simulink model "LINEFOLLOW_90_DATA_READING"  (R2023a)
settings: Solver=FixedStepDiscrete  StartTime=0.0  StopTime=250  FixedStep=0.01  RelTol=1e-3
model workspace (MAT data in the model file):
  data = 0
undefined symbols (not defined in the file or in its folder): axleLength, InputPWM, ticksPerRot, wheelR, WheelSpeed
libraries: mobileRoboticsTrainingLib x7, simulink_extras x1
settings Model: SimulationMode=accelerator  PacingRate=18  Creator=nuvitdemirtas  LastModifiedBy=nuvitdemirtas

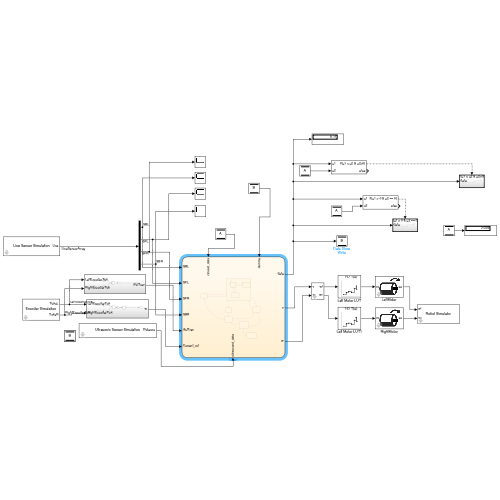
[thumbnail: Simulink's stored preview of the top-level diagram]
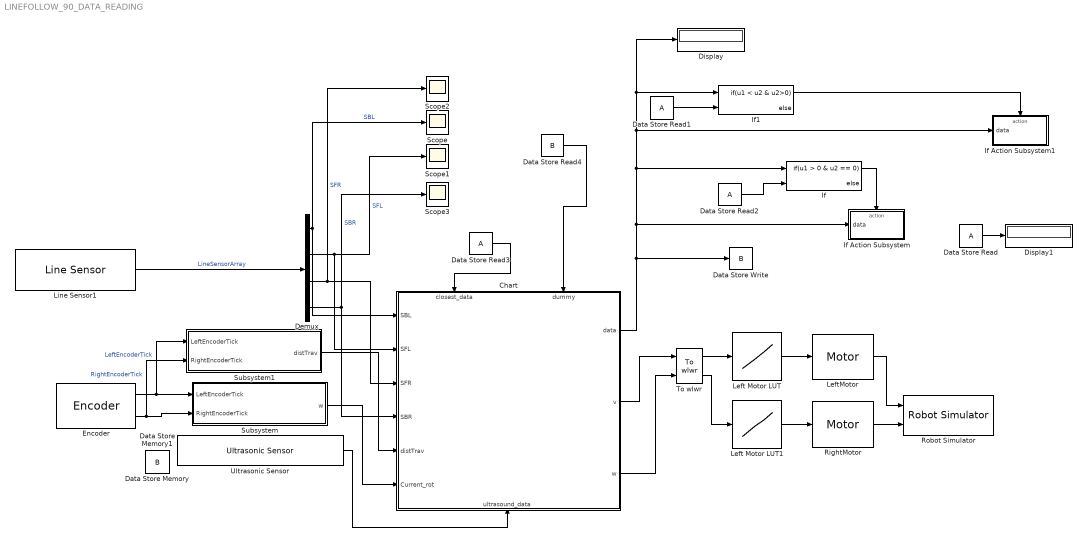
== system LINEFOLLOW_90_DATA_READING ==
  Chart : Stateflow chart  TreatAsAtomicUnit=on
      settings: PortSchema="{\"entries\":[{\"content\":{\"sides\":[{\"content\":{\"connectorIds\":[\"In5\",\"In3\",\"In2\",\"In4\",\"In7\",\"In6\"]},\"type\":\"ConnectorPlacement.EquallySpacedRectSide\",\"uuid\":\"3b08c9f5-f3e7-4190-8c9e-e5c4b273b76c\"},{\"content\":{\"connectorIds\":[\"Out3\",\"Out2\",\"Out1\"],\"side\":\"RIGHT\"},\"type\":\"ConnectorPlacement.EquallySpacedRectSide\",\"uuid\":\"91158a50-9984-4409-9676-111dc7610217\"},{\"content\":{\"connectorIds\":[\"In8\",\"In9\"],\"side\":\"TOP\"},\"type\":\"ConnectorPlacement.EquallySpacedRectSide\",\"uuid\":\"e43f7616-6a00-4e82-aaba-e999a0c0a235\"},{\"content\":{\"connectorIds\":[\"In1\"],\"side\":\"BOTTOM\"},\"type\":\"ConnectorPlacement.EquallySpacedRectSide\",\"uuid\":\"5780565f-9fed-471c-a43c-eef749218091\"}]},\"type\":\"ConnectorPlacement.EquallySpacedConnector\",\"uuid\":\"4b7d5f21-cf1e-4123-a6bd-16491044a199\"}],\"packageUris\":[\"http://schema.mathworks.com/mf0/Connector/R2020b\"],\"version\":\"1.0\"}"
  Data Store Read{,1..3} (4 alike) : DataStoreRead  IndexOptions=Index vector (dialog)  Indices=1  OutputSizes=1
  Data Store Read4 : DataStoreRead  DataStoreName=B  IndexOptions=Index vector (dialog)  Indices=1  OutputSizes=1
  Data Store Write : DataStoreWrite  DataStoreName=B  IndexOptions=Index vector (dialog)  Indices=1  OutputSizes=1
  Data Store Memory : DataStoreMemory  WriteAfterWriteMsg=warning  ShowAdditionalParam=off
  Data Store Memory1 : DataStoreMemory  DataStoreName=B  WriteAfterWriteMsg=warning  ShowAdditionalParam=off
  Demux : Demux
  Display : Display
  Display1 : Display
  Encoder : mobileRoboticsTrainingLib/Encoder  axleLength=axleLength  wheelR=wheelR  ticksPerRot=ticksPerRot
      settings: SourceProductName=Mobile Robotics Training Library
  If : If  NumInputs=2  IfExpression=u1 > 0 & u2 == 0
  If Action Subsystem : Subsystem  TreatAsAtomicUnit=on
  If Action Subsystem1 : Subsystem  TreatAsAtomicUnit=on
  If1 : If  NumInputs=2  IfExpression=u1 < u2 & u2>0
  Left Motor LUT : Lookup_n-D  NumberOfTableDimensions=1  BreakpointsForDimension1=WheelSpeed  Table=InputPWM  InterpMethod=Nearest  ExtrapMethod=Clip  InternalRulePriority=Speed  RndMeth=Simplest
  Left Motor LUT1 : Lookup_n-D  NumberOfTableDimensions=1  BreakpointsForDimension1=WheelSpeed  Table=InputPWM  InterpMethod=Nearest  ExtrapMethod=Clip  InternalRulePriority=Speed  RndMeth=Simplest
  LeftMotor : mobileRoboticsTrainingLib/Motor  motorPlant=wheelMotorModel  sensorType=Speed
      settings: SourceProductName=Mobile Robotics Training Library
  Line Sensor1 : mobileRoboticsTrainingLib/Line Sensor  mapVariable=mapForSim  envVal=1  lineVal=0  sensOff=[0.0643 0.0354; 0.0675 0.005; 0.0675 -0.005; 0.0643 -0.0354]
      link override Switch: Threshold=0
      settings: SourceProductName=Mobile Robotics Training Library
  RightMotor : mobileRoboticsTrainingLib/Motor  motorPlant=wheelMotorModel  sensorType=Speed
      settings: SourceProductName=Mobile Robotics Training Library
  Robot Simulator : mobileRoboticsTrainingLib/Robot Simulator  Priority=99  mapVar=mapForSim  startX=1.0088  startY=3.1003  startTheta=90  axleLength=axleLength  wheelR=wheelR
  Scope{,1..3} (4 alike) : Scope
  Subsystem : Subsystem
  Subsystem1 : Subsystem
  To wlwr : mobileRoboticsTrainingLib/To wlwr  axleLength=0.1  wheelR=0.05
  Ultrasonic Sensor : mobileRoboticsTrainingLib/Ultrasonic Sensor  mapVar=mapForSim  maxSenRange=4  minSenRange=0.02  senRes=0.003  sensOff=[0.1 0]
      settings: SourceProductName=Mobile Robotics Training Library
  wires:
  RightMotor/1 -> Robot Simulator/2
  LeftMotor/1 -> Robot Simulator/1
  To wlwr/2 -> Left Motor LUT1/1
  To wlwr/1 -> Left Motor LUT/1
  Chart/1(w) -> To wlwr/2
  Ultrasonic Sensor/1 -> Chart/1(ultrasound_data)
  Demux/4 -> Scope3/1, Chart/4(SBR)  "SBR"
  Encoder/2 -> Subsystem1/2(RightEncoderTick), Subsystem/2(RightEncoderTick)  "RightEncoderTick"
  Left Motor LUT1/1 -> RightMotor/1
  Demux/2 -> Chart/3(SFL), Scope1/1  "SFL"
  Demux/1 -> Scope/1, Chart/5(SBL)  "SBL"
  Chart/2(v) -> To wlwr/1
  Subsystem/1(w) -> Chart/6(Current_rot)
  Left Motor LUT/1 -> LeftMotor/1
  Demux/3 -> Chart/2(SFR), Scope2/1  "SFR"
  Encoder/1 -> Subsystem1/1(LeftEncoderTick), Subsystem/1(LeftEncoderTick)  "LeftEncoderTick"
  Line Sensor1/1 -> Demux/1  "LineSensorArray"
  Subsystem1/1(distTrav) -> Chart/7(distTrav)
  Chart/3(data) -> Data Store Write/1, Display/1, If1/1, If Action Subsystem1/1(data), If/1, If Action Subsystem/1(data)
  Data Store Read/1 -> Display1/1
  If/1 -> If Action Subsystem/Action
  Data Store Read1/1 -> If1/2
  If1/1 -> If Action Subsystem1/Action
  Data Store Read2/1 -> If/2
  Data Store Read3/1 -> Chart/8(closest_data)
  Data Store Read4/1 -> Chart/9(dummy)

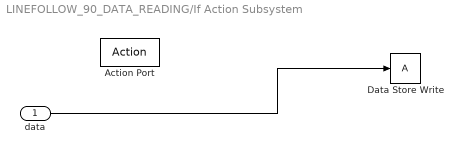
== system LINEFOLLOW_90_DATA_READING/If Action Subsystem ==
  data : Inport
  Action Port : ActionPort  ActionPortLabel=if(u1 > 0 & u2 == 0)
  Data Store Write : DataStoreWrite  IndexOptions=Index vector (dialog)  Indices=1  OutputSizes=1
  wires:
  data/1 -> Data Store Write/1

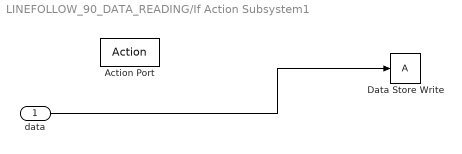
== system LINEFOLLOW_90_DATA_READING/If Action Subsystem1 ==
  data : Inport
  Action Port : ActionPort  ActionPortLabel=if(u1 < u2 & u2>0)
  Data Store Write : DataStoreWrite  IndexOptions=Index vector (dialog)  Indices=1  OutputSizes=1
  wires:
  data/1 -> Data Store Write/1

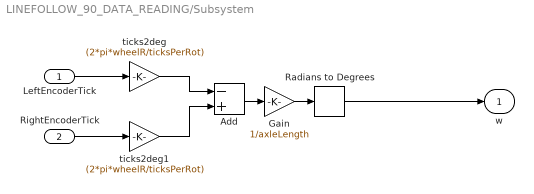
== system LINEFOLLOW_90_DATA_READING/Subsystem ==
  LeftEncoderTick : Inport
  RightEncoderTick : Inport  Port=2
  Add : Sum  Inputs=-+
  Gain : Gain  Gain=1/axleLength
  Radians to Degrees : simulink_extras/Transformations/Radians to Degrees
  ticks2deg : Gain  Gain=(2*pi*wheelR/ticksPerRot)
  ticks2deg1 : Gain  Gain=(2*pi*wheelR/ticksPerRot)
  w : Outport
  wires:
  Add/1 -> Gain/1
  ticks2deg/1 -> Add/1
  RightEncoderTick/1 -> ticks2deg1/1
  LeftEncoderTick/1 -> ticks2deg/1
  ticks2deg1/1 -> Add/2
  Radians to Degrees/1 -> w/1
  Gain/1 -> Radians to Degrees/1

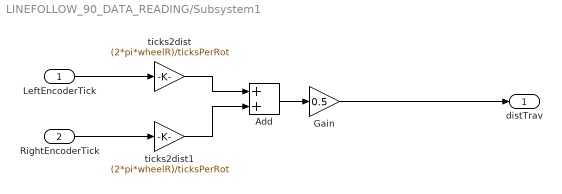
== system LINEFOLLOW_90_DATA_READING/Subsystem1 ==
  LeftEncoderTick : Inport
  RightEncoderTick : Inport  Port=2
  Add : Sum
  Gain : Gain  Gain=0.5
  ticks2dist : Gain  Gain=(2*pi*wheelR)/ticksPerRot
  ticks2dist1 : Gain  Gain=(2*pi*wheelR)/ticksPerRot
  distTrav : Outport
  wires:
  LeftEncoderTick/1 -> ticks2dist/1
  RightEncoderTick/1 -> ticks2dist1/1
  ticks2dist/1 -> Add/1
  ticks2dist1/1 -> Add/2
  Add/1 -> Gain/1
  Gain/1 -> distTrav/1

== stateflow chart LINEFOLLOW_90_DATA_READING/Chart ==
  state LINE_FOLLOW
    state perfect
      entry:
      v = 0.075;
      w = 0;
    state CORRECT_right
      entry:
      w = -1;
      v = 0.075;
    state CORRECT_left
      entry:
      w = 1;
      v = 0.075;
    (default) -> perfect
    perfect -> CORRECT_right [order 1] : [SFR == 0 && SFL ==1]
    CORRECT_right -> perfect : [SFR == 0 && SFL ==0]
    CORRECT_left -> perfect : [SFR == 0 && SFL ==0]
    perfect -> CORRECT_left [order 2] : [SFR == 1 && SFL ==0]
  state L_90
    entry:
    v= 0;
    w =  1;
  state a80_rot
    entry:
    v=0;
    w = 1;
    w_ref = Current_rot +175;
  state stop_measure
    entry:
    v = 0.05;
    w = 0;
    distRef = distTrav+0.07
  state stopping_distance
    entry:
    v= 0;
  state reverse
    entry:
    v = -0.05;
    w = 0;
    data = ultrasound_data;
    distRef = distTrav-0.07
    exit:
    v = 0
    data=ultrasound_data;
  state TREASURE_FOUND
    entry:
    v = 0;
    w = 0;
  (default) -> LINE_FOLLOW
  LINE_FOLLOW -> L_90 [order 1] : [SBR ==1 && SBL ==0 ]
  L_90 -> LINE_FOLLOW : [SFR == 0 && SFL ==0]
  LINE_FOLLOW -> a80_rot [order 3] : [SBR ==1 && SBL ==1 && SFL ==1 && SFR == 1 && ultrasound_data==0]
  stopping_distance -> L_90 [order 1] : [SBR ==1 && SBL ==1 && SFL ==1 && SFR == 1 && ultrasound_data==0]
  LINE_FOLLOW -> stop_measure [order 2] : [SBR ==0 && SBL ==0 && SFL ==0 && SFR == 0]
  a80_rot -> LINE_FOLLOW : [Current_rot>=w_ref  ]
  stop_measure -> stopping_distance : [distTrav >= distRef]
  stopping_distance -> a80_rot [order 2] : [[SBR ==0 && SBL ==0 && SFL ==0 && SFR == 0 && ultrasound_data==0]]
  reverse -> a80_rot [order 1] : [distTrav <= distRef]
  stopping_distance -> reverse [order 3] : [(ultrasound_data>0)]
  reverse -> TREASURE_FOUND [order 2] : [data<= closest_data+ 0.05 && data>= closest_data-0.05 && data>0 && (closest_data~= dummy) ]
  data: ultrasound_data input; w output; SFR input; SFL input; SBR input; SBL input; v output; Current_rot input; w_ref local; distTrav input; distRef local; data output; closest_data input; dummy input
